simulink model "autonomy"  (R2018b)
settings: Solver=VariableStepAuto  StartTime=0.0  StopTime=inf  RelTol=1e-3
undefined symbols (not defined in the file or in its folder): AltDesiredMeters, AltSwitch, PitchDesiredDegrees, PitchSwitch, RollDesiredDegrees, RollSwitch, YawDesiredDegrees, YawSwitch
libraries: robotlib x3
settings Model: Creator=amav  LastModifiedBy=zlacey

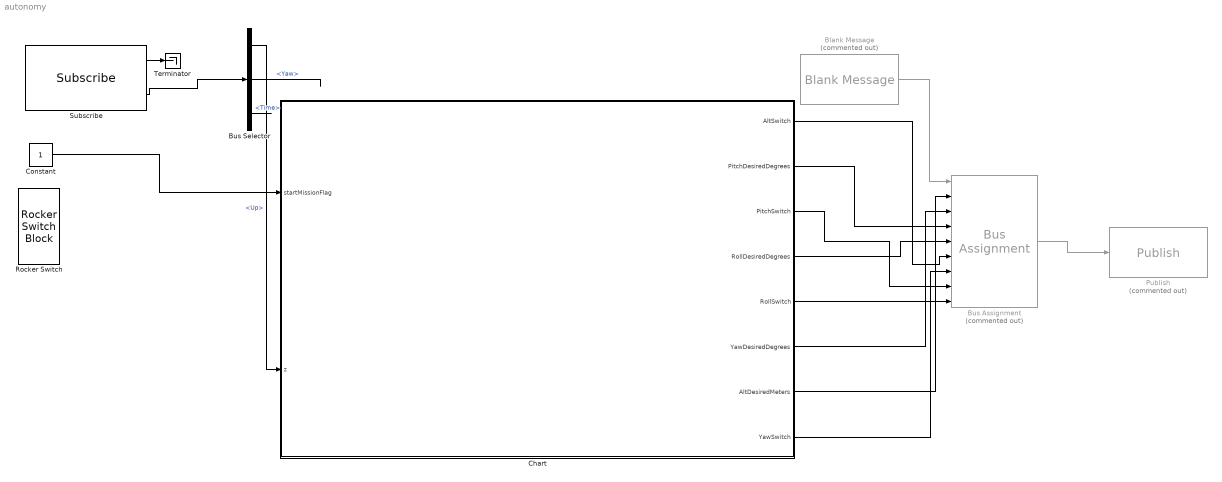
== system autonomy ==
  Blank Message : robotlib/Blank Message  Commented=on  messageClass=Message  entityType=terpcopter_msgs/ayprCmd  messageType=terpcopter_msgs/ayprCmd  SampleTime=inf
      settings: SourceProductBaseCode=RO
  Bus Assignment : BusAssignment  Commented=on  AssignedSignals=AltDesiredMeters,YawDesiredDegrees,PitchDesiredDegrees,RollDesiredDegrees,AltSwitch,YawSwitch,PitchSwitch,RollSwitch
  Bus Selector : BusSelector  OutputSignals=Up,Yaw,Time
  Chart : Stateflow chart  TreatAsAtomicUnit=on
  Constant : Constant
  Publish : robotlib/Publish  Commented=on  topicSource=Specify your own  topic=/ayprCmd  messageType=terpcopter_msgs/ayprCmd  messageQueueLength=1
      settings: SourceProductBaseCode=RO
  Rocker Switch : RockerSwitchBlock  WebBlockId=23
      settings: Values={{'Off', 'On'}, [0 1]}
  Subscribe : robotlib/Subscribe  topicSource=Select from ROS network  topic=/stateEstimate  messageType=terpcopter_msgs/stateEstimate  sampleTime=0.1  messageQueueLength=1
      settings: SourceProductBaseCode=RO
  Terminator : Terminator
  wires:
  Subscribe/2 -> Bus Selector/1
  Subscribe/1 -> Terminator/1
  Bus Selector/1 -> Chart/2(z)  "<Up>"
  Constant/1 -> Chart/1(startMissionFlag)
  Chart/7(AltDesiredMeters) -> Bus Assignment/2
  Chart/6(YawDesiredDegrees) -> Bus Assignment/3
  Chart/2(PitchDesiredDegrees) -> Bus Assignment/4
  Chart/4(RollDesiredDegrees) -> Bus Assignment/5
  Chart/1(AltSwitch) -> Bus Assignment/6
  Chart/8(YawSwitch) -> Bus Assignment/7
  Chart/3(PitchSwitch) -> Bus Assignment/8
  Chart/5(RollSwitch) -> Bus Assignment/9
  Bus Assignment/1 -> Publish/1
  Bus Selector/3 -> ?  "<Time>"
  Blank Message/1 -> Bus Assignment/1
  Bus Selector/2 -> ?  "<Yaw>"

== stateflow chart autonomy/Chart ==
  state InitializeAndStart
    entry:
    % aypr cmds
    AltSwitch = 0;
    YawSwitch = 0;
    PitchSwitch = 0;
    RollSwitch = 0;
    AltDesiredMeters = 0;
    YawDesiredDegrees = 0;
    PitchDesiredDegrees = 0;
    RollDesiredDegrees = 0;
  state TakeoffBehavior
    entry:
    zd = 1; %desired altitude (meters)
    takeoffAltThresh = 0.1; % z-zd must be less than this threshold (meters)
    maxAltSafety = 5; % maximum altitude safety condition (meters)
    during:
    AltSwitch = 1;
    YawSwitch = 0;
    PitchSwitch = 0;
    RollSwitch = 0;
    AltDesiredMeters = zd; % desired altitude cmd (meters)
  state HoverBehavior
    entry:
    zd = 1.5; % desired
    timeDesired = 1000; % desired hover time (seconds)
    AltDesiredMeters = zd; % desired altitude (meters)
  state LandBehavior
    entry:
  (default) -> InitializeAndStart
  InitializeAndStart -> TakeoffBehavior : [startMissionFlag == 1]
  TakeoffBehavior -> HoverBehavior : [abs(z-AltDesiredMeters) <= takeoffAltThresh || z >= maxAltSafety]{zd=1.25}
  HoverBehavior -> LandBehavior : [duration(abs(z-zd) <= 0.25)>= timeDesired]
  data: startMissionFlag input; z input; maxAltSafety local double; zd local double =0; takeoffAltThresh local; timeDesired local; AltSwitch output; PitchDesiredDegrees output; PitchSwitch output; RollDesiredDegrees output; RollSwitch output; YawDesiredDegrees output; AltDesiredMeters output; YawSwitch output
